simulink model "ClarkTransformationMatrix"  (R2022a)
settings: Solver=VariableStepAuto  StartTime=0.0  StopTime=10.0  RelTol=1e-3
settings Model: Creator=jff_1  LastModifiedBy=jff_1

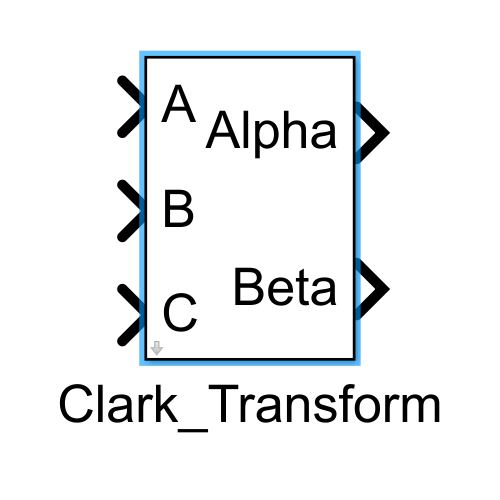
[thumbnail: Simulink's stored preview of the top-level diagram]
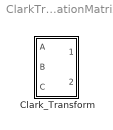
== system ClarkTransformationMatrix ==
  Clark_Transform : Subsystem
      mask help:
      | Clark坐标变换（abc → αβ）
      |
      | 采用幅值不变形式（2/3 系数）
      | 适用于三相对称、无零序分量的系统
      mask Help: 现代永磁同步电机控制原理及MATLAB仿真P5
      mask DialogControl ParameterGroupVar Prompt: 参数
      mask Display:
      | % 输入端口标签（1~3）
      | port_label('input',1,'A');
      | port_label('input',2,'B');
      | port_label('input',3,'C');
      | 
      | % 输出端口标签（1~2）
      | port_label('output',1,'Alpha');
      | port_label('output',2,'Beta');

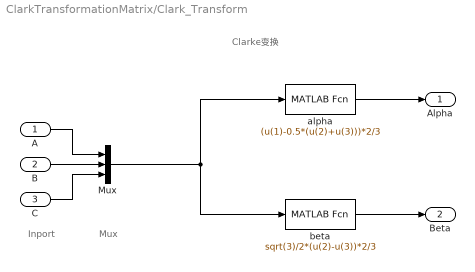
== system ClarkTransformationMatrix/Clark_Transform ==
  note: Clarke变换
  note: Inport
  note: Mux
  A : Inport
  B : Inport  Port=2
  C : Inport  Port=3
  Mux : Mux  Inputs=3
  alpha : MATLABFcn  MATLABFcn=(u(1)-0.5*(u(2)+u(3)))*2/3
  beta : MATLABFcn  MATLABFcn=sqrt(3)/2*(u(2)-u(3))*2/3
  Alpha : Outport
  Beta : Outport  Port=2
  wires:
  Mux/1 -> beta/1, alpha/1
  beta/1 -> Beta/1
  alpha/1 -> Alpha/1
  C/1 -> Mux/3
  B/1 -> Mux/2
  A/1 -> Mux/1
